simulink model "RDataGeneration"  (R2017b)
settings: Solver=ode5  StartTime=0.0  StopTime=1000  FixedStep=0.0025  RelTol=1e-3  AbsTol=1e-6
libraries: DABLib x4
settings Model: Creator=davidlaredorazo  LastModifiedBy=dlaredo
settings DataIOCC: SaveFormat=Array  SignalLoggingSaveFormat=ModelDataLogs
settings OptimizationCC: BlockReduction=off  BooleanDataType=off
settings DebuggingCC: SaveWithParameterizedLinksMsg=none  UnderspecifiedInitializationDetection=Classic  MergeDetectMultiDrivingBlocksExec=none  SignalResolutionControl=TryResolveAllWithWarning  MultiTaskDSMMsg=warning  MultiTaskCondExecSysMsg=none
settings HardwareCC: TargetUnknown=on
settings ModelReferenceCC: PropagateSignalLabelsOutOfModel=off
settings GRTTargetCC: TargetLangStandard=C89/C90 (ANSI)  CombineOutputUpdateFcns=off  GRTInterface=on

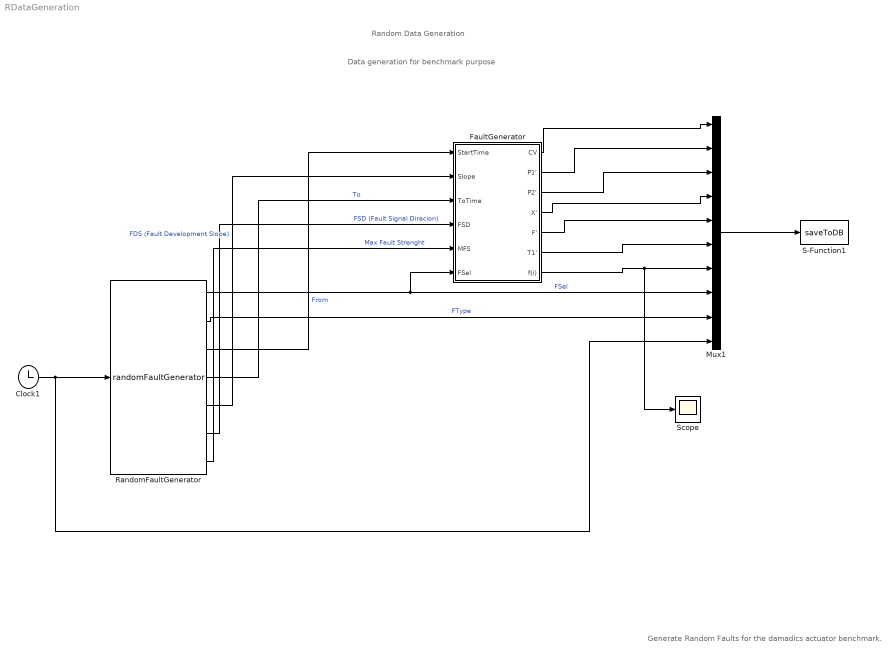
== system RDataGeneration ==
  note: Data generation for benchmark purpose
  note: Random Data Generation
  note: Generate Random Faults for the damadics actuator benchmark.
  Clock1 : Clock
  FaultGenerator : Subsystem
  Mux1 : Mux  Inputs=10
  RandomFaultGenerator : S-Function  FunctionName=randomFaultGenerator  SFunctionDeploymentMode=off  EnableBusSupport=off
      mask Display:
      | port_label('input', 1, 'realClock');
      | port_label('output', 1, 'Fsel');
      | port_label('output', 2, 'Ftype');
      | port_label('output', 3, 'From');
      | port_label('output', 4, 'To');
      | port_label('output', 5, 'FDS');
      | port_label('output', 6, 'FSD');
      | port_label('output', 7, 'MFS');
  S-Function1 : S-Function  FunctionName=saveToDB  SFunctionDeploymentMode=off  EnableBusSupport=off
  Scope : Scope
  wires:
  FaultGenerator/1(CV) -> Mux1/1
  FaultGenerator/3(P2') -> Mux1/3
  FaultGenerator/4(X') -> Mux1/4
  FaultGenerator/5(F') -> Mux1/5
  FaultGenerator/6(T1') -> Mux1/6
  Clock1/1 -> Mux1/10, RandomFaultGenerator/1
  RandomFaultGenerator/1 -> FaultGenerator/6(FSel), Mux1/8  "FSel"
  RandomFaultGenerator/2 -> Mux1/9  "FType"
  FaultGenerator/2(P1') -> Mux1/2
  FaultGenerator/7(f(i)) -> Scope/1, Mux1/7
  Mux1/1 -> S-Function1/1
  RandomFaultGenerator/3 -> FaultGenerator/1(StartTime)  "From"
  RandomFaultGenerator/4 -> FaultGenerator/3(ToTime)  "To"
  RandomFaultGenerator/5 -> FaultGenerator/2(Slope)  "FDS (Fault Development Slope)"
  RandomFaultGenerator/6 -> FaultGenerator/4(FSD)  "FSD (Fault Signal Direcion)"
  RandomFaultGenerator/7 -> FaultGenerator/5(MFS)  "Max Fault Strenght"

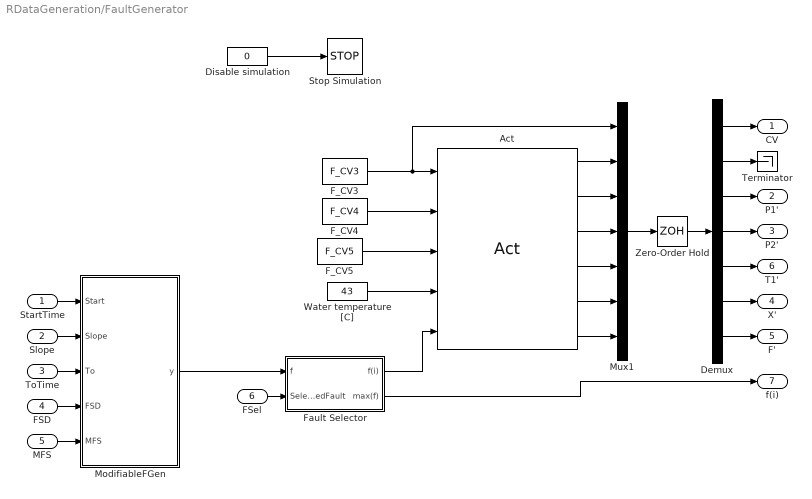
== system RDataGeneration/FaultGenerator ==
  StartTime : Inport
  Slope : Inport  Port=2
  ToTime : Inport  Port=3
  FSD : Inport  Port=4
  MFS : Inport  Port=5
  FSel : Inport  Port=6
  Act : DABLib/Act  Dist=off
  Demux : Demux  Outputs=7
  Disable simulation : Constant  Value=0
  F_CV3 : DABLib/DGen/F_CV3  A=0.25  f=0.01  c=0.5
  F_CV4 : DABLib/DGen/F_CV4  A=175000  f=0.1  c=3500000
  F_CV5 : DABLib/DGen/F_CV5  A=26000  f=1/pi  c=2600000
  Fault Selector : Subsystem  AncestorBlock=DABLib/DGen/Fault Selector
  ModifiableFGen : Subsystem
  Mux1 : Mux  Inputs=7
  Stop Simulation : Stop
  Terminator : Terminator
  "Water temperature [C] " : Constant  Value=43
  Zero-Order Hold : ZeroOrderHold
  CV : Outport  InitialOutput=0
  P1' : Outport  Port=2  InitialOutput=0
  P2' : Outport  Port=3  InitialOutput=0
  X' : Outport  Port=4  InitialOutput=0
  F' : Outport  Port=5  InitialOutput=0
  T1' : Outport  Port=6  InitialOutput=0
  f(i) : Outport  Port=7  InitialOutput=0
  wires:
  Act/6 -> Mux1/7
  Zero-Order Hold/1 -> Demux/1
  Demux/1 -> CV/1
  Demux/4 -> P2'/1
  ModifiableFGen/1(y) -> Fault Selector/1(f)
  Act/2 -> Mux1/3
  Demux/2 -> Terminator/1
  Disable simulation/1 -> Stop Simulation/1
  Demux/3 -> P1'/1
  Demux/7 -> F'/1
  Act/3 -> Mux1/4
  Mux1/1 -> Zero-Order Hold/1
  F_CV5/1 -> Act/3
  Act/1 -> Mux1/2
  "Water temperature [C] "/1 -> Act/4
  Act/5 -> Mux1/6
  Act/4 -> Mux1/5
  Fault Selector/1(f(i)) -> Act/5
  Demux/6 -> X'/1
  Demux/5 -> T1'/1
  Fault Selector/2(max(f)) -> f(i)/1
  F_CV3/1 -> Mux1/1, Act/1
  F_CV4/1 -> Act/2
  StartTime/1 -> ModifiableFGen/1(Start)
  Slope/1 -> ModifiableFGen/2(Slope)
  FSD/1 -> ModifiableFGen/4(FSD)
  ToTime/1 -> ModifiableFGen/3(To)
  MFS/1 -> ModifiableFGen/5(MFS)
  FSel/1 -> Fault Selector/2(SelectedFault)

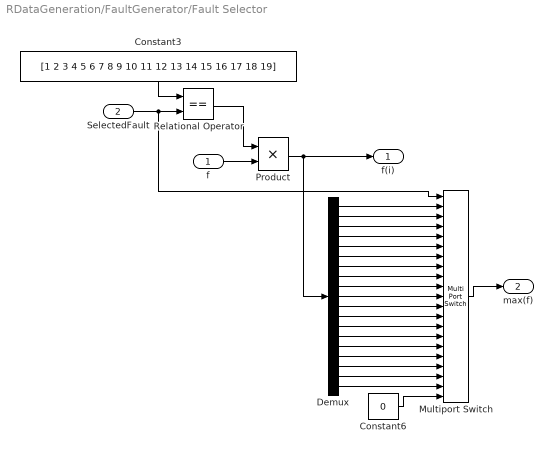
== system RDataGeneration/FaultGenerator/Fault Selector ==
  f : Inport
  SelectedFault : Inport  Port=2
  Constant3 : Constant  Value=[1 2 3 4 5 6 7 8 9 10 11 12 13 14 15 16 17 18 19]
  Constant6 : Constant  Value=0
  Demux : Demux  Outputs=19
  Multiport Switch : MultiPortSwitch  Inputs=20  SaturateOnIntegerOverflow=on  InputSameDT=on
  Product : Product  SaturateOnIntegerOverflow=on  RndMeth=Zero  InputSameDT=on  OutDataTypeStr=Inherit: Same as first input
  Relational Operator : RelationalOperator  Operator===  RndMeth=Nearest  InputSameDT=on
  f(i) : Outport  InitialOutput=0
  max(f) : Outport  Port=2  InitialOutput=0
  wires:
  Demux/3 -> Multiport Switch/4
  Demux/4 -> Multiport Switch/5
  Demux/5 -> Multiport Switch/6
  Demux/6 -> Multiport Switch/7
  Demux/7 -> Multiport Switch/8
  Demux/8 -> Multiport Switch/9
  Demux/9 -> Multiport Switch/10
  Demux/10 -> Multiport Switch/11
  Demux/11 -> Multiport Switch/12
  Demux/12 -> Multiport Switch/13
  Demux/13 -> Multiport Switch/14
  Demux/14 -> Multiport Switch/15
  Demux/15 -> Multiport Switch/16
  Demux/16 -> Multiport Switch/17
  Demux/17 -> Multiport Switch/18
  Demux/18 -> Multiport Switch/19
  Demux/19 -> Multiport Switch/20
  Multiport Switch/1 -> max(f)/1
  Constant6/1 -> Multiport Switch/21
  Product/1 -> Demux/1, f(i)/1
  SelectedFault/1 -> Multiport Switch/1, Relational Operator/2
  Demux/1 -> Multiport Switch/2
  Demux/2 -> Multiport Switch/3
  f/1 -> Product/2
  Constant3/1 -> Relational Operator/1
  Relational Operator/1 -> Product/1

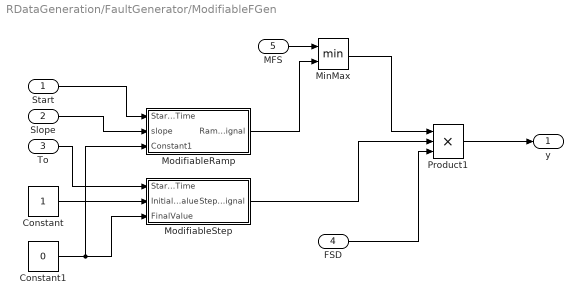
== system RDataGeneration/FaultGenerator/ModifiableFGen ==
  Start : Inport
  Slope : Inport  Port=2
  To : Inport  Port=3
  FSD : Inport  Port=4
  MFS : Inport  Port=5
  Constant : Constant
  Constant1 : Constant  Value=0
  MinMax : MinMax  Inputs=2
  ModifiableRamp : Subsystem
  ModifiableStep : Subsystem
  Product1 : Product  Inputs=3  SaturateOnIntegerOverflow=on  RndMeth=Zero  InputSameDT=on  OutDataTypeStr=Inherit: Same as first input
  y : Outport  InitialOutput=0
  wires:
  FSD/1 -> Product1/3
  ModifiableRamp/1(RampSignal) -> MinMax/2
  Product1/1 -> y/1
  Constant/1 -> ModifiableStep/2(InitialValue)
  Slope/1 -> ModifiableRamp/2(slope)
  Start/1 -> ModifiableRamp/1(StartingTime)
  ModifiableStep/1(StepSignal) -> Product1/2
  MinMax/1 -> Product1/1
  To/1 -> ModifiableStep/1(StartingTime)
  Constant1/1 -> ModifiableStep/3(FinalValue), ModifiableRamp/3(Constant1)
  MFS/1 -> MinMax/1

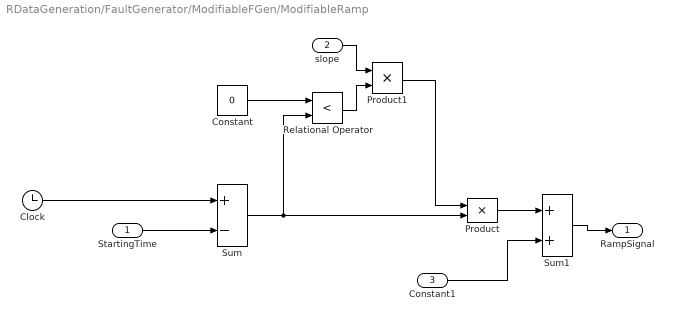
== system RDataGeneration/FaultGenerator/ModifiableFGen/ModifiableRamp ==
  StartingTime : Inport
  slope : Inport  Port=2
  Constant1 : Inport  Port=3
  Clock : Clock
  Constant : Constant  Value=0
  Product : Product  SaturateOnIntegerOverflow=on  RndMeth=Zero  InputSameDT=on  OutDataTypeStr=Inherit: Same as first input
  Product1 : Product
  Relational Operator : RelationalOperator  Operator=<  OutDataTypeStr=boolean  RndMeth=Simplest
  Sum : Sum  Inputs=+-  SaturateOnIntegerOverflow=on  InputSameDT=on  OutDataTypeStr=Inherit: Same as first input
  Sum1 : Sum  SaturateOnIntegerOverflow=on  InputSameDT=on  OutDataTypeStr=Inherit: Same as first input
  RampSignal : Outport
  wires:
  Sum/1 -> Relational Operator/2, Product/2
  Constant1/1 -> Sum1/2
  Product/1 -> Sum1/1
  Clock/1 -> Sum/1
  Sum1/1 -> RampSignal/1
  StartingTime/1 -> Sum/2
  Constant/1 -> Relational Operator/1
  slope/1 -> Product1/1
  Relational Operator/1 -> Product1/2
  Product1/1 -> Product/1

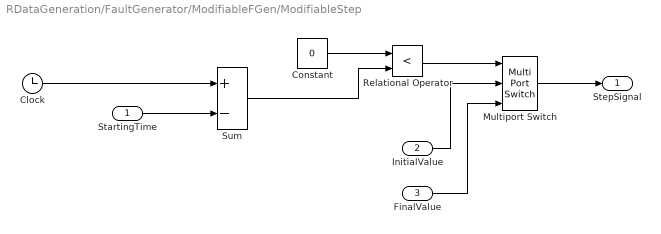
== system RDataGeneration/FaultGenerator/ModifiableFGen/ModifiableStep ==
  StartingTime : Inport
  InitialValue : Inport  Port=2
  FinalValue : Inport  Port=3
  Clock : Clock
  Constant : Constant  Value=0
  Multiport Switch : MultiPortSwitch  DataPortOrder=Zero-based contiguous  Inputs=2
  Relational Operator : RelationalOperator  Operator=<  OutDataTypeStr=boolean  RndMeth=Simplest
  Sum : Sum  Inputs=+-  SaturateOnIntegerOverflow=on  InputSameDT=on  OutDataTypeStr=Inherit: Same as first input
  StepSignal : Outport
  wires:
  Constant/1 -> Relational Operator/1
  Sum/1 -> Relational Operator/2
  Clock/1 -> Sum/1
  StartingTime/1 -> Sum/2
  Relational Operator/1 -> Multiport Switch/1
  FinalValue/1 -> Multiport Switch/3
  InitialValue/1 -> Multiport Switch/2
  Multiport Switch/1 -> StepSignal/1
